simulink model "Microinverter_Paper_with_control_experimental_10-31-18"  (R2018a)
settings: Solver=FixedStepDiscrete  StartTime=0.0  StopTime=0.3  RelTol=1e-3
undefined symbols (not defined in the file): sigbuilder_block
libraries: powerlib x42, simulink x4, powerlib_meascontrol x2, re_lib x1
settings Model: Creator=jasil  LastModifiedBy=mstruong
settings SFSimCC: SimUseLocalCustomCode=on
settings RTWCC: RTWUseLocalCustomCode=on
settings CodeAppCC: StateflowObjectComments=on

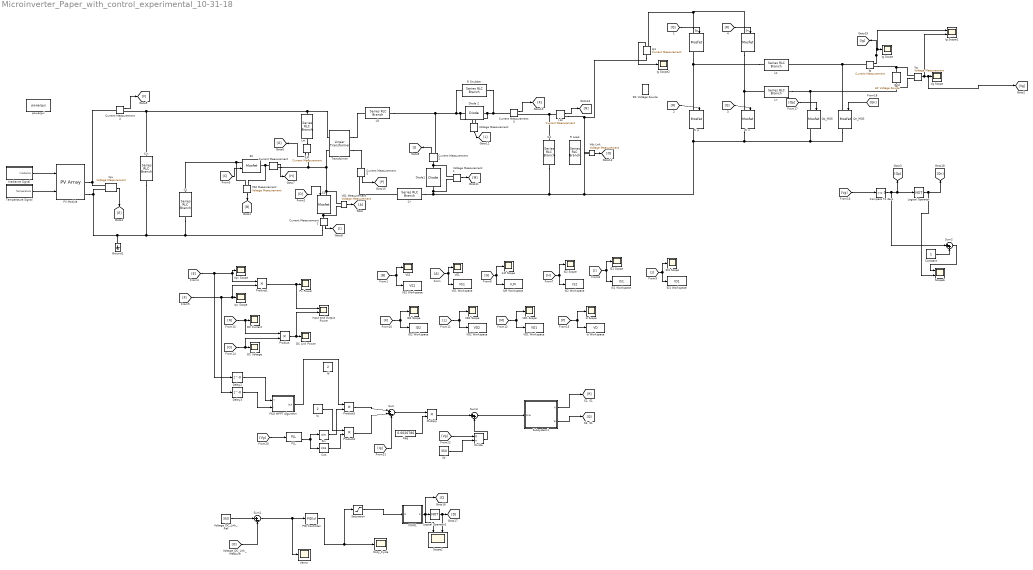
== system Microinverter_Paper_with_control_experimental_10-31-18 ==
  Cc : powerlib/Elements/Series RLC Branch  LConnTagsString=__new0  RConnTagsString=__new0  BranchType=RC  Resistance=0.000001  Inductance=1e-3  SetiL0=off  InitialCurrent=0  Capacitance=2.2e-6  Setx0=off  InitialVoltage=0  Measurements=None
  Cd : powerlib/Elements/Series RLC Branch  LConnTagsString=__new0  RConnTagsString=__new0  BranchType=RC  Resistance=0.000001  Inductance=1e-3  SetiL0=off  InitialCurrent=0  Capacitance=1e-6  Setx0=off  InitialVoltage=0  Measurements=None
  Cin : powerlib/Elements/Series RLC Branch  LConnTagsString=__new0  RConnTagsString=__new0  BranchType=RC  Resistance=0.000001  Inductance=1e-3  SetiL0=off  InitialCurrent=0  Capacitance=1e-3  Setx0=off  InitialVoltage=0  Measurements=Branch voltage
  Compare To Zero : simulink/Logic and Bit Operations/Compare To Zero  relop=>=  OutDataTypeStr=boolean
  Constant : Constant
  Cos : Trigonometry  Operator=cos
  Cr : powerlib/Elements/Series RLC Branch  LConnTagsString=__new0  RConnTagsString=__new0  BranchType=RC  Resistance=0.000001  Inductance=1e-3  SetiL0=off  InitialCurrent=0  Capacitance=2.4e-6  Setx0=off  InitialVoltage=0  Measurements=None
  Current Measurement{,1..5} (6 alike) : powerlib/Measurements/Current Measurement  PhasorSimulation=off  OutputType=Complex  PSBequivalent=0
  DC Current : Scope
  DC Link Power : Scope
  DC Voltage : Scope
  DC Voltage Source : powerlib/Electrical Sources/DC Voltage Source  Amplitude=350  Measurements=None
  Delay2 : Delay  DelayLength=0  SampleTime=0.001
  Delay3 : Delay  DelayLength=0  SampleTime=0.001
  Diode 2 : powerlib/Power Electronics/Diode  Ron=1  Lon=0  Vf=0.8  IC=0  UseSnubber=0  Rs=inf  Cs=0  Measurements=off
  Diode1 : powerlib/Power Electronics/Diode  Ron=0.01  Lon=0  Vf=0.8  IC=0  UseSnubber=0  Rs=inf  Cs=0  Measurements=off
  Divide : Product  Inputs=*/
  Duty_Cycle : Scope
  Grid : powerlib/Electrical Sources/AC Voltage Source  Amplitude=311.126  Phase=0  Frequency=60  SampleTime=0  Measurements=None  BusType=swing  Pref=10e3  Qref=0  Qmin=-inf  Qmax=+inf
  Ground1 : powerlib/Elements/Ground  LConnTagsString=a
  I dc : powerlib/Measurements/Current Measurement  PhasorSimulation=off  OutputType=Complex  PSBequivalent=0
  ID1 Scope : Scope
  ID1 Workspace : ToWorkspace  VariableName=ID1  SaveFormat=Timeseries  SampleTime=-1
  ID2 Scope : Scope
  ID2 Workspace : ToWorkspace  VariableName=ID2  SaveFormat=Timeseries  SampleTime=-1
  ILM Workspace : ToWorkspace  VariableName=ILM  SaveFormat=Timeseries  SampleTime=-1
  IS1 Scope : Scope
  IS1 Workspace : ToWorkspace  VariableName=IS1  SaveFormat=Timeseries  SampleTime=-1
  IS2 Scope : Scope
  IS2 Workspace : ToWorkspace  VariableName=IS2  SaveFormat=Timeseries  SampleTime=-1
  Id : Constant  Value=2
  Ig : powerlib/Measurements/Current Measurement  PhasorSimulation=off  OutputType=Complex  PSBequivalent=0
  Ig Scope : Scope
  Ig Scope1 : Scope  NumInputPorts=2
  Ig Scope2 : Scope
  Ig1 : powerlib/Measurements/Current Measurement  PhasorSimulation=off  OutputType=Complex  PSBequivalent=0
  Input and Output Power : Scope  NumInputPorts=2
  Ipv Scope : Scope
  Iq : Constant  Value=2
  "Irradiance Signal " : Subsystem  Tag=STV Subsys  LoadFcn=sigbuilder_block('load');  StartFcn=sigbuilder_block('start');  StopFcn=sigbuilder_block('stop');  ClipboardFcn=sigbuilder_block('clipboard');  mask(Sigbuilder block){tuvar=[0:10]}
      mask help: Simulink:masks:SigbuilderBlock_MD
      mask init:
      | if ~strcmp(get_param(bdroot(gcbh),'SimulationStatus'),'stopped') tuvar = sigbuilder_block('maskInit'); end
      settings: CopyFcn=sigbuilder_block('copy');  DeleteFcn=sigbuilder_block('delete');  ModelCloseFcn=sigbuilder_block('modelClose');  PreSaveFcn=sigbuilder_block('preSave');  PauseFcn=sigbuilder_block('pause');  ContinueFcn=sigbuilder_block('continue');  NameChangeFcn=sigbuilder_block('namechange');  OpenFcn=sigbuilder_block('open',[6 30 1012.5 447.75 ]);  CloseFcn=sigbuilder_block('close');
      mask Display: plot(0, 0, 100, 100,[2, 2, 32, 32, 2], [68, 8, 8, 68, 68],[32, 2], [38, 38], [32, 19, 2],[53, 60, 44], [32, 17, 17, 2],[16, 16, 31, 31]);txt = getActiveGroup(gcbh);text(2, 100, txt,'verticalAlignment', 'top');
  Is Scope : Scope
  Is Workspace : ToWorkspace  VariableName=VD  SaveFormat=Timeseries  SampleTime=-1
  Kpg : Constant  Value=0.0026786
  Llk : powerlib/Elements/Series RLC Branch  LConnTagsString=__new0  RConnTagsString=__new0  BranchType=RL  Resistance=0.000001  Inductance=2.6e-6  SetiL0=off  InitialCurrent=0  Capacitance=1e-6  Setx0=off  InitialVoltage=0  Measurements=None
  Lm : powerlib/Elements/Series RLC Branch  LConnTagsString=__new0  RConnTagsString=__new0  BranchType=RL  Resistance=0.000001  Inductance=20e-6  SetiL0=off  InitialCurrent=0  Capacitance=1e-6  Setx0=off  InitialVoltage=0  Measurements=None
  Ln : powerlib/Elements/Series RLC Branch  LConnTagsString=__new0  RConnTagsString=__new0  BranchType=RL  Resistance=0.000001  Inductance=15e-3  SetiL0=off  InitialCurrent=0  Capacitance=1e-6  Setx0=off  InitialVoltage=0  Measurements=None
  Logical Operator : Logic  Operator=NOT  AllPortsSameDT=off  OutDataTypeStr=boolean
  Logical Operator2 : Logic  Operator=NOT  AllPortsSameDT=off  OutDataTypeStr=boolean
  Lp : powerlib/Elements/Series RLC Branch  LConnTagsString=__new0  RConnTagsString=__new0  BranchType=RL  Resistance=0.000001  Inductance=15e-3  SetiL0=off  InitialCurrent=0  Capacitance=1e-6  Setx0=off  InitialVoltage=0  Measurements=None
  Multiply : Product
  P&O MPPT Algorithm : MATLAB Function  TreatAsAtomicUnit=on
  PID Controller : simulink/Continuous/PID Controller  Controller=PID  TimeDomain=Discrete-time  SampleTime=-1  IntegratorMethod=Forward Euler  FilterMethod=Forward Euler  Form=Parallel  UseFilter=on  ControllerParametersSource=internal  P=50  I=1  D=0  N=100  InitialConditionSource=internal  InitialConditionForIntegrator=0  InitialConditionForFilter=0  ExternalReset=none  LimitOutput=off  UpperSaturationLimit=inf  LowerSaturationLimit=-inf  LinearizeAsGain=on  AntiWindupMode=none  Kb=1  TrackingMode=off  Kt=1  PParamMin=[]  PParamMax=[]  IParamMin=[]  IParamMax=[]  DParamMin=[]  DParamMax=[]  NParamMin=[]  NParamMax=[]  KbParamMin=[]  KbParamMax=[]  KtParamMin=[]  KtParamMax=[]  POutMin=[]  POutMax=[]  IOutMin=[]  IOutMax=[]  DOutMin=[]  DOutMax=[]  NOutMin=[]  NOutMax=[]  KbOutMin=[]  KbOutMax=[]  KtOutMin=[]  KtOutMax=[]  IntegratorOutMin=[]  IntegratorOutMax=[]  FilterOutMin=[]  FilterOutMax=[]  SumOutMin=[]  SumOutMax=[]  SumI1OutMin=[]  SumI1OutMax=[]  SumI2OutMin=[]  SumI2OutMax=[]  SumI3OutMin=[]  SumI3OutMax=[]  SumDOutMin=[]  SumDOutMax=[]  SaturationOutMin=[]  SaturationOutMax=[]  IntegratorContinuousStateAttributes=''  IntegratorStateMustResolveToSignalObject=off  IntegratorRTWStateStorageClass=Auto  FilterContinuousStateAttributes=''  FilterStateMustResolveToSignalObject=off  FilterRTWStateStorageClass=Auto  DifferentiatorICPrevScaledInput=0  DifferentiatorOutMin=[]  DifferentiatorOutMax=[]  FilterDiffOutCoefMin=[]  FilterDiffOutCoefMax=[]  SumDenOutMin=[]  SumDenOutMax=[]  SumNumOutMin=[]  SumNumOutMax=[]  ReciprocalOutMin=[]  ReciprocalOutMax=[]  DivideOutMin=[]  DivideOutMax=[]  TunerSelectOption=Transfer Function Based (PID Tuner App)
  PLL : powerlib_meascontrol/PLL/PLL  Fmin=45  Par_Init=[0, 60]  ParK=[180, 3200, 1]  TcD=1e-4  MaxRateChangeFreq=12  FilterCutOffFreq=25  Ts=1e-6  AGC=on
      settings: SourceProductName=Simscape Power Systems  SourceProductBaseCode=PS
  PV Module : re_lib/Solar/PV Array  Npar=1  Nser=2  PlotType=array @ 25 deg.C & specified irradiances  S_vec="[ 1000  500  100 ]"  Temp_C_vec="[ 45 25  ]"  ModuleName=User-defined  PlotWhenSelected=off  Pm=179.9805  Ncell=36  Voc=24.06  Isc=9.77  Vm=19.67  Im=9.15  beta_Voc_pc=-0.28  alpha_Isc_pc=+0.04  beta_Voc=-0.067368  alpha_Isc=0.003908  IL=9.8911  I0=1.3829e-11  nI=0.95443  Rsh=60.4787  Rs=0.18212  BAL=off  Tc=1e-6  Tfilter=5e-5
  PWM1 : Subsystem
  Product{,1,3..4} (4 alike) : Product
  Pv Power : Scope
  Qn_MOS : powerlib/Power Electronics/Mosfet  Ron=0.1  Lon=0  Rd=0.01  Vfd=0  IC=0  Rs=1e5  Cs=inf  Measurements=on
  Qp_MOS : powerlib/Power Electronics/Mosfet  Ron=0.1  Lon=0  Rd=0.01  Vfd=0  IC=0  Rs=1e5  Cs=inf  Measurements=on
  R Load : powerlib/Elements/Series RLC Branch  LConnTagsString=__new0  RConnTagsString=__new0  BranchType=R  Resistance=695  Inductance=1e-3  SetiL0=off  InitialCurrent=0  Capacitance=1e-6  Setx0=off  InitialVoltage=0  Measurements=None
  R Snubber : powerlib/Elements/Series RLC Branch  LConnTagsString=__new0  RConnTagsString=__new0  BranchType=R  Resistance=1e6  Inductance=1e-3  SetiL0=off  InitialCurrent=0  Capacitance=1e-6  Setx0=off  InitialVoltage=0  Measurements=None
  S' n : powerlib/Power Electronics/Mosfet  Ron=0.1  Lon=0  Rd=0.01  Vfd=0  IC=0  Rs=1e5  Cs=inf  Measurements=on
  S' p : powerlib/Power Electronics/Mosfet  Ron=0.1  Lon=0  Rd=0.01  Vfd=0  IC=0  Rs=1e5  Cs=inf  Measurements=on
  S1 : powerlib/Power Electronics/Mosfet  Ron=5.6e-3  Lon=0  Rd=0.01  Vfd=1.3  IC=0  Rs=1e6  Cs=inf  Measurements=off
  S2 : powerlib/Power Electronics/Mosfet  Ron=5.6e-3  Lon=0  Rd=0.01  Vfd=1.3  IC=0  Rs=1e5  Cs=inf  Measurements=off
  Saturation : Saturate  UpperLimit=1  LowerLimit=0
  Scope2 : Scope  NumInputPorts=2
  Scope6 : Scope  NumInputPorts=2
  Sin : Trigonometry
  Sn : powerlib/Power Electronics/Mosfet  Ron=0.1  Lon=0  Rd=0.01  Vfd=0  IC=0  Rs=1e5  Cs=inf  Measurements=on
  Sp : powerlib/Power Electronics/Mosfet  Ron=0.1  Lon=0  Rd=0.01  Vfd=0  IC=0  Rs=1e5  Cs=inf  Measurements=on
  Subsystem1 : Subsystem
  Sum : Sum  Inputs=|++-
  Sum1 : Sum  Inputs=|+-
  Sum2 : Sum  Inputs=|++
  Sum3 : Sum  Inputs=|++
  Temperature Signal : Subsystem  Tag=STV Subsys  LoadFcn=sigbuilder_block('load');  StartFcn=sigbuilder_block('start');  StopFcn=sigbuilder_block('stop');  ClipboardFcn=sigbuilder_block('clipboard');  mask(Sigbuilder block){tuvar=[0:10]}
      mask help: Simulink:masks:SigbuilderBlock_MD
      mask init:
      | if ~strcmp(get_param(bdroot(gcbh),'SimulationStatus'),'stopped') tuvar = sigbuilder_block('maskInit'); end
      settings: CopyFcn=sigbuilder_block('copy');  DeleteFcn=sigbuilder_block('delete');  ModelCloseFcn=sigbuilder_block('modelClose');  PreSaveFcn=sigbuilder_block('preSave');  PauseFcn=sigbuilder_block('pause');  ContinueFcn=sigbuilder_block('continue');  NameChangeFcn=sigbuilder_block('namechange');  OpenFcn=sigbuilder_block('open',[6 30 1012.5 447.75 ]);  CloseFcn=sigbuilder_block('close');
      mask Display: plot(0, 0, 100, 100,[2, 2, 32, 32, 2], [68, 8, 8, 68, 68],[32, 2], [38, 38], [32, 19, 2],[53, 60, 44], [32, 17, 17, 2],[16, 16, 31, 31]);txt = getActiveGroup(gcbh);text(2, 100, txt,'verticalAlignment', 'top');
  Transformer : powerlib/Elements/Linear Transformer  UNITS=SI  NominalPower=[ 25 100e3 ]  winding1=[6.36 0 0]  winding2=[26.87 0 0]  ThreeWindings=off  winding3=[3.15e+05 3.969e+07 6316.9]  RmLm=[1e6 Inf]  Measurements=None  DataType=on
  VD1 Scope : Scope
  VD1 Workspace : ToWorkspace  VariableName=VD1  SaveFormat=Timeseries  SampleTime=-1
  VD2 Scope : Scope
  VD2 Workspace : ToWorkspace  VariableName=VD2  SaveFormat=Timeseries  SampleTime=-1
  VS1 : Scope
  VS1 Measurement : powerlib/Measurements/Voltage Measurement  PhasorSimulation=off  OutputType=Complex  PSBequivalent=0
  VS1 Workspace : ToWorkspace  VariableName=VS1  SaveFormat=Timeseries  SampleTime=-1
  VS2 : Scope
  VS2 Measurement : powerlib/Measurements/Voltage Measurement  PhasorSimulation=off  OutputType=Complex  PSBequivalent=0
  VS2 Workspace : ToWorkspace  VariableName=VS2  SaveFormat=Timeseries  SampleTime=-1
  Vd : Constant  Value=350
  Vdc Link : powerlib/Measurements/Voltage Measurement  PhasorSimulation=off  OutputType=Complex  PSBequivalent=0
  "Verror " : Scope
  Vg : powerlib/Measurements/Voltage Measurement  PhasorSimulation=off  OutputType=Complex  PSBequivalent=0
  Vg Scope : Scope
  Voltage Measurement : powerlib/Measurements/Voltage Measurement  PhasorSimulation=off  OutputType=Complex  PSBequivalent=0
  Voltage Measurement1 : powerlib/Measurements/Voltage Measurement  PhasorSimulation=off  OutputType=Complex  PSBequivalent=0
  Voltage_DC_Link_Ref : Constant  Value=350
  Vpv : powerlib/Measurements/Voltage Measurement  PhasorSimulation=off  OutputType=Complex  PSBequivalent=0
  Vpv Scope : Scope
  iLM : powerlib/Measurements/Current Measurement  PhasorSimulation=off  OutputType=Complex  PSBequivalent=0
  iLM Scope : Scope
  powergui : powerlib/powergui  Priority=1  SimulationMode=Discrete  SampleTime=9e-8  frequency=60  Iterations=50  frequencyindice=0  Pbase=100e6  ErrMax=1e-4  UnitsV=kV  UnitsW=MW  buscounter=0  FunctionMessages=off  echomessages=off  EnableUseOfTLC=off  CurrentSourceSwitches=off  DisableSnubberDevices=off  DisableRonSwitches=off  DisableVfSwitches=off  DisplayEquations=off  SolverType=Tustin/Backward Euler (TBE)  Interpol=off  ExternalGateDelay=off  methode=off  Ts=100  x0status=blocks  SPID=on  SwTol=0  HookPort=off  RestoreLinks=warning  ResistiveCurrentMeasurement=off  Frange=[0:2:500]  Ylog=off  Xlog=on  ShowGrid=off  save=off  variable=ZData  structure=0  ZoomFFT=off  StartTime=0.0  cycles=1  DisplayStyle=1  fundamental=60  FreqAxis=off  MaxFrequency=1000  frequencyindicesteady=1  RmsSteady=1  display=off
  wires:
  [M] -> VD1 Workspace/1, VD1 Scope/1
  Vdc Link/1 -> [O]
  "Irradiance Signal "/1(Irradiance) -> PV Module/1
  [O] -> Product/2, DC Voltage/1
  VS2 Measurement/1 -> [B]
  Current Measurement1/1 -> [I]
  Vpv/1 -> [E]
  Voltage Measurement/1 -> [L]
  Voltage Measurement1/1 -> [M]
  [C] -> S2/1
  Current Measurement2/1 -> [J]
  [L] -> VD2 Workspace/1, VD2 Scope/1
  [J] -> ID1 Workspace/1, ID1 Scope/1
  [E] -> Delay2/1, Vpv Scope/1, Product1/1
  [F] -> Delay3/1, Product1/2, Ipv Scope/1
  Current Measurement/1 -> [H]
  [A] -> VS1 Workspace/1, VS1/1
  [D] -> S1/1
  [I] -> IS1 Workspace/1, IS1 Scope/1
  [B] -> VS2 Workspace/1, VS2/1
  iLM/1 -> [G]
  Product/1 -> Input and Output Power/2, DC Link Power/1
  [G] -> iLM Scope/1, ILM Workspace/1
  Delay3/1 -> P&O MPPT Algorithm/2(I)
  [K] -> ID2 Workspace/1, ID2 Scope/1
  Product1/1 -> Input and Output Power/1, Pv Power/1
  [H] -> IS2 Workspace/1, IS2 Scope/1
  VS1 Measurement/1 -> [A]
  [N] -> Product/1, DC Current/1
  Temperature Signal/1(Temperature) -> PV Module/2
  Delay2/1 -> P&O MPPT Algorithm/1(V)
  [P] -> Is Workspace/1, Is Scope/1
  Current Measurement4/1 -> [F]
  I dc/1 -> [N]
  Current Measurement3/1 -> [K]
  Current Measurement5/1 -> [P]
  PID Controller/1 -> Saturation/1, Duty_Cycle/1
  Logical Operator2/1 -> Scope2/2, [D]
  PWM1/1(S) -> Scope2/1, [C], Logical Operator2/1
  Voltage_DC_Link_Ref/1 -> Sum1/1
  [O] -> Sum1/2
  Sum1/1 -> PID Controller/1, "Verror "/1
  Saturation/1 -> PWM1/1(D)
  Logical Operator/1 -> Scope6/2, [Qn]
  Vg/1 -> Ig Scope1/2, [Vg], Vg Scope/1
  [Qn] -> Qn_MOS/1
  [R] -> Sn/1
  [Q] -> Sp/1
  [Q] -> S' n/1
  [Qp] -> Qp_MOS/1
  [Vg] -> Compare To Zero/1
  Ig1/1 -> Ig Scope2/1
  Ig/1 -> [Ig], Ig Scope1/1, Ig Scope/1
  [R] -> S' p/1
  Subsystem1/1(A) -> [R]
  Subsystem1/2(B) -> [Q]
  Constant/1 -> Sum2/2
  Compare To Zero/1 -> Sum2/1, [Qp], Logical Operator/1
  Sum2/1 -> Scope6/1
  [Vg] -> PLL/1
  PLL/2 -> Sin/1, Cos/1
  Sin/1 -> Product3/2
  P&O MPPT Algorithm/1(Iout) -> Product3/1
  Cos/1 -> Product4/2
  Product3/1 -> Sum/1
  Product4/1 -> Sum/2
  [Ig] -> Sum/3
  Sum/1 -> Multiply/1
  Kpg/1 -> Multiply/2
  Multiply/1 -> Sum3/1
  [Vg] -> Divide/1
  Vd/1 -> Divide/2
  Divide/1 -> Sum3/2
  Iq/1 -> Product4/1
  Sum3/1 -> Subsystem1/1(Sine)
  connections:
  Current Measurement1/RConn1 -- Ground1/LConn1 -- Vpv/LConn2 -- PV Module/RConn2 -- Cin/RConn1 -- Cc/RConn1
  Llk/RConn1 -- R Snubber/LConn1 -- Voltage Measurement/LConn2 -- Diode 2/LConn1 -- Current Measurement2/RConn1
  VS1 Measurement/LConn2 -- Current Measurement1/LConn1 -- S1/RConn1
  Qp_MOS/RConn1 -- Cr/RConn1 -- Voltage Measurement1/LConn2 -- Diode1/LConn1 -- Cd/RConn1 -- Vdc Link/LConn2 -- S' p/RConn1 -- S' n/RConn1 -- Qn_MOS/RConn1
  S2/LConn1 -- VS2 Measurement/LConn1 -- Cc/LConn1
  iLM/RConn1 -- S1/LConn1 -- VS1 Measurement/LConn1 -- Transformer/LConn2 -- Current Measurement/RConn1
  Cd/LConn1 -- I dc/LConn1 -- Current Measurement3/RConn1
  S2/RConn1 -- VS2 Measurement/LConn2 -- Current Measurement/LConn1
  Lm/RConn1 -- iLM/LConn1
  Cr/LConn1 -- Current Measurement5/RConn1
  I dc/RConn1 -- Ig1/LConn1 -- Vdc Link/LConn1
  Lm/LConn1 -- Cin/LConn1 -- Current Measurement4/RConn1 -- Transformer/LConn1
  PV Module/RConn1 -- Vpv/LConn1 -- Current Measurement4/LConn1
  Diode 2/RConn1 -- Voltage Measurement/LConn1 -- R Snubber/RConn1 -- Current Measurement3/LConn1
  Diode1/RConn1 -- Voltage Measurement1/LConn1 -- Current Measurement2/LConn1
  Ig/RConn1 -- Grid/RConn1 -- Vg/LConn1
  Lp/LConn1 -- Sp/RConn1 -- S' p/LConn1
  Vg/LConn2 -- Grid/LConn1 -- Qp_MOS/LConn1 -- Ln/RConn1
  Ln/LConn1 -- S' n/LConn1 -- Sn/RConn1
  Sp/LConn1 -- Sn/LConn1 -- Ig1/RConn1
  Lp/RConn1 -- Ig/LConn1 -- Qn_MOS/LConn1
  Transformer/RConn2 -- Current Measurement5/LConn1
  Transformer/RConn1 -- Llk/LConn1

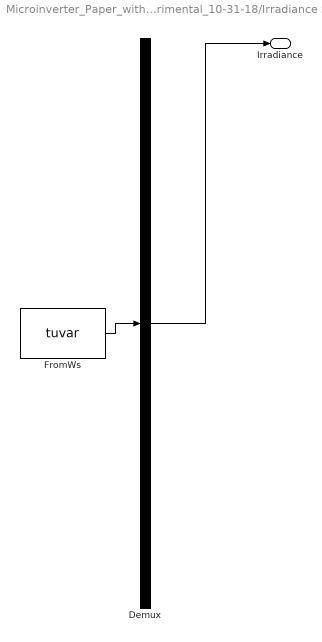
== system Microinverter_Paper_with_control_experimental_10-31-18/Irradiance Signal  ==
  Demux : Demux  Tag=STV Demux  Outputs=1
  FromWs : FromWorkspace  Tag=STV FromWs  VariableName=tuvar  SampleTime=0
      SigBuilderData=|
      | common.afterFinalStr = 'Extrapolate'
      | common.sampleTime = 0
      | dataSet.timeRange = [0 0.3]
      | dataSet.name = 'Group 1'
      | sbobj.Groups.Name = 'Group 1'
      | sbobj.Groups.Signals.Name = 'Irradiance'
      | sbobj.Groups.Signals.XData = [0 0.1 0.1 0.2 0.2 0.3]
      | sbobj.Groups.Signals.YData = [1000 1000 1000 1000 1000 1000]
      | sbobj.Groups.TimeRange = [0 0.3]
  Irradiance : Outport  Tag=STV Outport
  wires:
  Demux/1 -> Irradiance/1
  FromWs/1 -> Demux/1

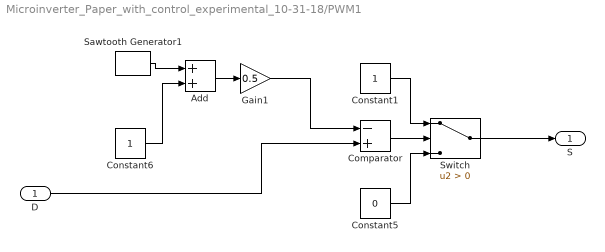
== system Microinverter_Paper_with_control_experimental_10-31-18/PWM1 ==
  D : Inport
  Add : Sum
  Comparator : Sum  Inputs=-+
  Constant1 : Constant
  Constant5 : Constant  Value=0
  Constant6 : Constant
  Gain1 : Gain  Gain=0.5
  Sawtooth Generator1 : powerlib_meascontrol/Pulse & Signal Generators/Sawtooth Generator  Freq=50000  Phase=180  Ts=0
      settings: SourceProductName=Simscape Electrical
  Switch : Switch  Criteria=u2 > Threshold
  S : Outport
  wires:
  Switch/1 -> S/1
  Constant1/1 -> Switch/1
  Comparator/1 -> Switch/2
  Constant6/1 -> Add/2
  Gain1/1 -> Comparator/1
  Constant5/1 -> Switch/3
  Sawtooth Generator1/1 -> Add/1
  Add/1 -> Gain1/1
  D/1 -> Comparator/2

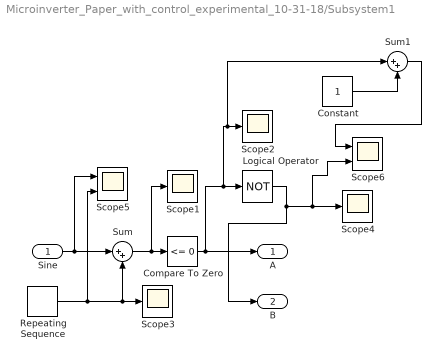
== system Microinverter_Paper_with_control_experimental_10-31-18/Subsystem1 ==
  Sine : Inport
  Compare To Zero : simulink/Logic and Bit Operations/Compare To Zero  relop=<=  OutDataTypeStr=boolean
  Constant : Constant
  Logical Operator : Logic  Operator=NOT  AllPortsSameDT=off  OutDataTypeStr=boolean
  Repeating Sequence : simulink/Sources/Repeating Sequence  rep_seq_t=[0 1/(4*16000) 3/(4*16000) 1/16000]  rep_seq_y=[0 1 -1 0]
  Scope{1..4} (4 alike) : Scope
  Scope5 : Scope  NumInputPorts=2
  Scope6 : Scope  NumInputPorts=2
  Sum : Sum  Inputs=|++
  Sum1 : Sum  Inputs=|++
  A : Outport
  B : Outport  Port=2
  wires:
  Logical Operator/1 -> Scope6/2, Scope4/1, B/1
  Sum/1 -> Scope1/1, Compare To Zero/1
  Repeating Sequence/1 -> Scope5/2, Scope3/1, Sum/2
  Sine/1 -> Scope5/1, Sum/1
  Compare To Zero/1 -> A/1, Sum1/1, Scope2/1, Logical Operator/1
  Constant/1 -> Sum1/2
  Sum1/1 -> Scope6/1

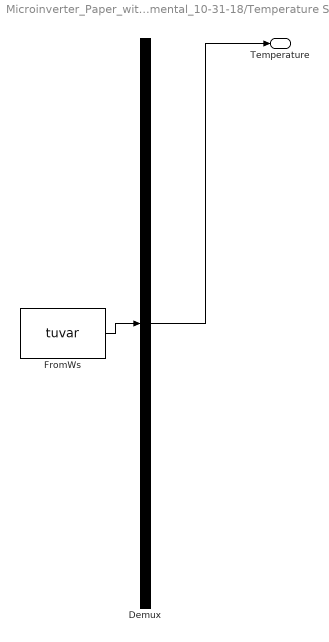
== system Microinverter_Paper_with_control_experimental_10-31-18/Temperature Signal ==
  Demux : Demux  Tag=STV Demux  Outputs=1
  FromWs : FromWorkspace  Tag=STV FromWs  VariableName=tuvar  SampleTime=0
      SigBuilderData=|
      | common.afterFinalStr = 'Extrapolate'
      | common.sampleTime = 0
      | dataSet.timeRange = [0 0.3]
      | dataSet.name = 'Group 1'
      | sbobj.Groups.Name = 'Group 1'
      | sbobj.Groups.Signals.Name = 'Temperature'
      | sbobj.Groups.Signals.XData = [0 0.1 0.1 0.2 0.2 0.3]
      | sbobj.Groups.Signals.YData = [25 25 25 25 25 25]
      | sbobj.Groups.TimeRange = [0 0.3]
  Temperature : Outport  Tag=STV Outport
  wires:
  Demux/1 -> Temperature/1
  FromWs/1 -> Demux/1

== matlab function Microinverter_Paper_with_control_experimental_10-31-18/P&O MPPT Algorithm ==
  data: V input; Iout output; I input
% function D = PandO(V, I)
% persistent p_prev;
% persistent v_prev;
% persistent d_prev; 
% 
% 
% if isempty(d_prev)
%     d_prev = 0.69;
%     v_prev = 24.06;
%     p_prev = 0;
% end
% 
% % Select the change in duty cycle
% delta_D = 0.001;
% 
% % Set local variables and calculate pv module power 
% Vn = V;
% In = I;
% Pn = Vn*In;
% 
% % Increase or decrease duty cycle based on conditions
% if ((Pn - p_prev) ~= 0)
%     if ((Pn - p_prev) > 0)
%         if ((Vn - v_prev) > 0)
%             D = d_prev - delta_D;
%         else
%             D = d_prev + delta_D;
%         end
%     else
%         if ((Vn - v_prev) > 0)
%             D = d_prev + delta_D;
%         else
%             D = d_prev - delta_D;
%         end        
%     end
% else
%     D = d_prev;
% end
% 
% % Update internal values
% d_prev = D;
% v_prev = Vn;
% p_prev = Pn;

function Iout = fcn(V,I)

persistent Vprev Pprev Iprev;

if isempty(Vprev)
    Vprev=30;
    Pprev=0;
    Iprev=0;
end

deltaI=0.1;

P = V * I;
    if (P>Pprev)
        if V > Vprev
            Iout = I + deltaI;
        else
            Iout = I - deltaI;
        end
    else
        if V > Vprev
            Iout = I - deltaI;
        else
            Iout = I + deltaI;
        end
    end
Vprev = V;
Pprev = P;
Iprev = I;

end
